simulink model "Simulink_with_unkown_parameters_case"  (R2020b)
settings: Solver=FixedStepAuto  StartTime=0.0  StopTime=50  FixedStep=0.001  MaxStep=0.01  RelTol=1e-9
values from neighbouring files (symbols this model uses):
  A0 = [30 3;3 30]    [Main_with_unkown_parameters_case.m]
  A1 = [30 3;3 30]    [Main_with_unkown_parameters_case.m]
  A2 = [10 1;1 10]    [Main_with_unkown_parameters_case.m]
  AE = blkdiag([0 pi/2;-pi/2 0],[0 pi/2;-pi/2 0])    [Main.m]    (also in Main_with_unkown_parameters_case.m)
  AM = blkdiag([0 1;-1 0],[0 1;-1 0])    [Main.m]    (also in Main_with_unkown_parameters_case.m)
  dq1_0 = [0;0]    [Main.m]    (also in Main_with_unkown_parameters_case.m)
  dq2_0 = [0;0]    [Main.m]    (also in Main_with_unkown_parameters_case.m)
  dq3_0 = [0;0]    [Main.m]    (also in Main_with_unkown_parameters_case.m)
  dq4_0 = [0;0]    [Main.m]    (also in Main_with_unkown_parameters_case.m)
  GammaE = blkdiag([1 0],[1 0])    [Main.m]    (also in Main_with_unkown_parameters_case.m)
  GammaM = blkdiag([1 0],[1 0])    [Main.m]    (also in Main_with_unkown_parameters_case.m)
  kapa = 100    [Main_with_unkown_parameters_case.m]
  Kd = 600    [Main.m]    (also in Main_with_unkown_parameters_case.m)
  Kp = 800    [Main.m]    (also in Main_with_unkown_parameters_case.m)
  l1 = 1.5    [Main.m]    (also in Main_with_unkown_parameters_case.m)
  l2 = 1.5    [Main.m]    (also in Main_with_unkown_parameters_case.m)
  M0 = [p1+p2+p4,p2;p2,p2+p5]+[2*p3,p3;p3,0]*cos(0)*0.5    [Main_with_unkown_parameters_case.m]
  N = 100    [Main_with_unkown_parameters_case.m]
  ON_OFF = 0    [Main.m]    (also in Main_with_unkown_parameters_case.m)
  p1 = m1*lc1^2+m2*l1^2+2*m2*l1*lc2^2+I1    (= 4.8375)    [Main.m]    (also in Main_with_unkown_parameters_case.m)
  p10 = 0    [Main.m]    (also in Main_with_unkown_parameters_case.m)
  p2 = m2*lc2^2+I2    (= 0.75)    [Main.m]    (also in Main_with_unkown_parameters_case.m)
  p3 = m2*l1*lc2    (= 1.125)    [Main.m]    (also in Main_with_unkown_parameters_case.m)
  p4 = 0    [Main.m]    (also in Main_with_unkown_parameters_case.m)
  p5 = 0    [Main.m]    (also in Main_with_unkown_parameters_case.m)
  p6 = (m1*lc1+m2*l1)*g    (= 23.544)    [Main.m]    (also in Main_with_unkown_parameters_case.m)
  p7 = m2*lc2*g    (= 7.3575)    [Main.m]    (also in Main_with_unkown_parameters_case.m)
  p8 = m2*lc2    (= 0.75)    [Main.m]    (also in Main_with_unkown_parameters_case.m)
  p9 = 0    [Main.m]    (also in Main_with_unkown_parameters_case.m)
  q1_0 = [-0.1;pi/3+0.2]    [Main.m]    (also in Main_with_unkown_parameters_case.m)
  q2_0 = [pi/2;2*pi/3]    [Main.m]    (also in Main_with_unkown_parameters_case.m)
  q3_0 = [pi-0.2;pi/3+0.2]    [Main.m]    (also in Main_with_unkown_parameters_case.m)
  q4_0 = [0.2;-pi/3-0.2]    [Main.m]    (also in Main_with_unkown_parameters_case.m)
  x1_0 = [0;0]    [Main.m]    (also in Main_with_unkown_parameters_case.m)
  x2_0 = [5;0]    [Main.m]    (also in Main_with_unkown_parameters_case.m)
  x3_0 = [5;3]    [Main.m]    (also in Main_with_unkown_parameters_case.m)
  x4_0 = [0;3]    [Main.m]    (also in Main_with_unkown_parameters_case.m)
(part 1 of 2)
settings Model: Creator=sokra  LastModifiedBy=sokra

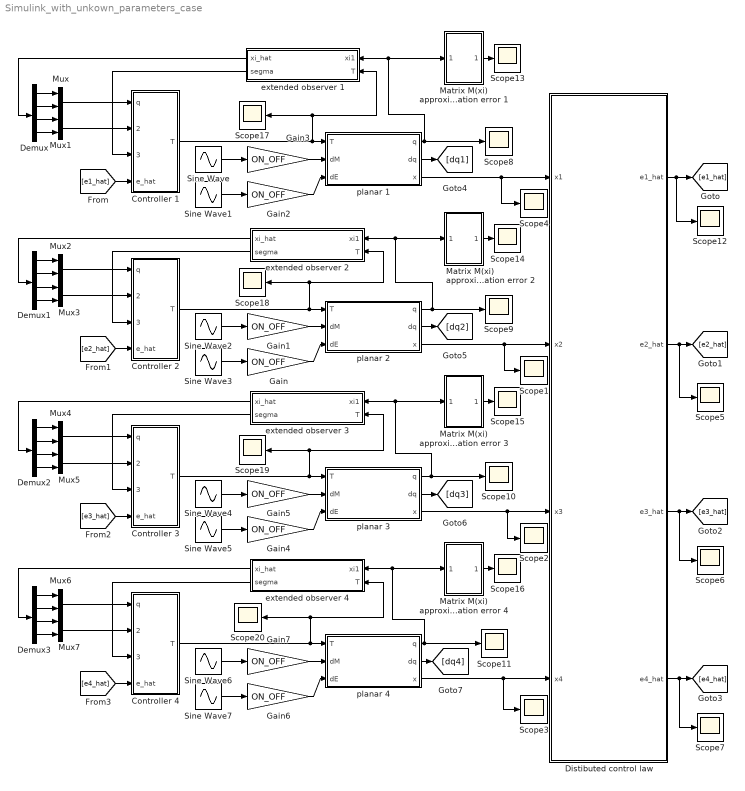
== system Simulink_with_unkown_parameters_case ==
  Controller 1 : Subsystem
  Controller 2 : Subsystem
  Controller 3 : Subsystem
  Controller 4 : Subsystem
  Demux{,1..3} (4 alike) : Demux
  Distibuted control law : MATLAB Function  TreatAsAtomicUnit=on
  Gain{,1..7} (8 alike) : Gain  Gain=ON_OFF
  Matrix M(xi) approximation error 1 : Subsystem
  Matrix M(xi) approximation error 2 : Subsystem
  Matrix M(xi) approximation error 3 : Subsystem
  Matrix M(xi) approximation error 4 : Subsystem
  Mux{,1..7} (8 alike) : Mux  Inputs=2
  Scope{1..20} (20 alike) : Scope
  Sine Wave{,2,4,6} (4 alike) : Sin  Amplitude=[1;1]  Frequency=[1;1]  SampleTime=0
  Sine Wave{1,3,5,7} (4 alike) : Sin  Amplitude=[1;1]/2  Frequency=[1;1]*pi/2  SampleTime=0
  extended observer 1 : Subsystem
  extended observer 2 : Subsystem
  extended observer 3 : Subsystem
  extended observer 4 : Subsystem
  planar 1 : Subsystem  mask{q_0=q1_0, dq_0=dq1_0, x0=x1_0}
  planar 2 : Subsystem  mask{q_0=q2_0, dq_0=dq2_0, x0=x2_0}
  planar 3 : Subsystem  mask{q_0=q3_0, dq_0=dq3_0, x0=x3_0}
  planar 4 : Subsystem  mask{q_0=q4_0, dq_0=dq4_0, x0=x4_0}
  wires:
  Controller 1/1(T) -> Scope17/1, extended observer 1/2(T), planar 1/1(T)
  planar 1/1(q) -> Scope8/1, Matrix M(xi) approximation error 1/1(xi1), extended observer 1/1(xi1)
  planar 2/1(q) -> Scope9/1, Matrix M(xi) approximation error 2/1(xi1), extended observer 2/1(xi1)
  Controller 2/1(T) -> planar 2/1(T), extended observer 2/2(T), Scope18/1
  Controller 3/1(T) -> extended observer 3/2(T), Scope19/1, planar 3/1(T)
  planar 3/1(q) -> Matrix M(xi) approximation error 3/1(xi1), extended observer 3/1(xi1), Scope10/1
  planar 4/1(q) -> Scope11/1, Matrix M(xi) approximation error 4/1(xi1), extended observer 4/1(xi1)
  Controller 4/1(T) -> extended observer 4/2(T), Scope20/1, planar 4/1(T)
  planar 1/3(x) -> Scope4/1, Distibuted control law/1(x1)
  planar 2/3(x) -> Scope1/1, Distibuted control law/2(x2)
  planar 3/3(x) -> Scope2/1, Distibuted control law/3(x3)
  planar 4/3(x) -> Scope3/1, Distibuted control law/4(x4)
  Distibuted control law/1(e1_hat) -> Scope12/1, [e1_hat]
  Distibuted control law/2(e2_hat) -> Scope5/1, [e2_hat]
  Distibuted control law/3(e3_hat) -> Scope6/1, [e3_hat]
  Distibuted control law/4(e4_hat) -> Scope7/1, [e4_hat]
  [e1_hat] -> Controller 1/4(e_hat)
  [e2_hat] -> Controller 2/4(e_hat)
  [e3_hat] -> Controller 3/4(e_hat)
  [e4_hat] -> Controller 4/4(e_hat)
  Gain/1 -> planar 2/3(dE)
  Gain1/1 -> planar 2/2(dM)
  Sine Wave2/1 -> Gain1/1
  Sine Wave3/1 -> Gain/1
  Sine Wave/1 -> Gain3/1
  Sine Wave1/1 -> Gain2/1
  Gain3/1 -> planar 1/2(dM)
  Sine Wave4/1 -> Gain5/1
  Sine Wave5/1 -> Gain4/1
  Gain5/1 -> planar 3/2(dM)
  Sine Wave6/1 -> Gain7/1
  Sine Wave7/1 -> Gain6/1
  Gain7/1 -> planar 4/2(dM)
  Gain6/1 -> planar 4/3(dE)
  Gain4/1 -> planar 3/3(dE)
  Gain2/1 -> planar 1/3(dE)
  planar 1/2(dq) -> [dq1]
  planar 2/2(dq) -> [dq2]
  planar 3/2(dq) -> [dq3]
  planar 4/2(dq) -> [dq4]
  extended observer 1/1(xi_hat) -> Demux/1
  Demux/2 -> Mux/2
  Demux/1 -> Mux/1
  Demux/3 -> Mux1/1
  Demux/4 -> Mux1/2
  Mux/1 -> Controller 1/1(q)
  Mux1/1 -> Controller 1/2(dq_hat)
  Demux1/2 -> Mux2/2
  Demux1/1 -> Mux2/1
  Demux1/4 -> Mux3/2
  Demux1/3 -> Mux3/1
  Demux2/3 -> Mux5/1
  Demux2/1 -> Mux4/1
  Demux2/4 -> Mux5/2
  Demux2/2 -> Mux4/2
  Demux3/3 -> Mux7/1
  Demux3/1 -> Mux6/1
  Demux3/4 -> Mux7/2
  Demux3/2 -> Mux6/2
  Mux2/1 -> Controller 2/1(q)
  Mux3/1 -> Controller 2/2(dq_hat)
  Mux4/1 -> Controller 3/1(q)
  Mux5/1 -> Controller 3/2(dq_hat)
  Mux6/1 -> Controller 4/1(q)
  Mux7/1 -> Controller 4/2(dq_hat)
  extended observer 4/1(xi_hat) -> Demux3/1
  extended observer 3/1(xi_hat) -> Demux2/1
  extended observer 2/1(xi_hat) -> Demux1/1
  extended observer 1/2(segma) -> Controller 1/3(segma)
  extended observer 2/2(segma) -> Controller 2/3(segma)
  extended observer 3/2(segma) -> Controller 3/3(segma)
  extended observer 4/2(segma) -> Controller 4/3(segma)
  Matrix M(xi) approximation error 1/1(error) -> Scope13/1
  Matrix M(xi) approximation error 2/1(error) -> Scope14/1
  Matrix M(xi) approximation error 3/1(error) -> Scope15/1
  Matrix M(xi) approximation error 4/1(error) -> Scope16/1

== system Simulink_with_unkown_parameters_case/Controller 1 ==
  q : Inport
  dq_hat : Inport  Port=2
  segma : Inport  Port=3
  e_hat : Inport  Port=4
  Compensator : Subsystem
  Gain1 : Gain  Gain=-Kd
  Gain2 : Gain  Gain=-Kp
  Gain3 : Gain  Gain=ON_OFF
  Gain4 : Gain  Gain=M0  Multiplication=Matrix(K*u)
  Jacobian matrix : Subsystem
  Product1 : Product  Multiplication=Matrix(*)
  Saturation : Saturate  UpperLimit=N  LowerLimit=-N
  Sum2 : Sum  Inputs=+-
  Sum5 : Sum  Inputs=+++
  Transpose : Math  Operator=transpose  SaturateOnIntegerOverflow=on
  T : Outport
  wires:
  dq_hat/1 -> Compensator/1(dq), Gain1/1
  Gain1/1 -> Sum5/3
  Sum5/1 -> Sum2/1
  Jacobian matrix/1(J(q)) -> Transpose/1
  Transpose/1 -> Compensator/2(J(q)), Gain2/1
  Gain2/1 -> Product1/1
  Product1/1 -> Sum5/2
  e_hat/1 -> Product1/2
  Compensator/1(ud) -> Gain3/1
  Gain3/1 -> Sum5/1
  q/1 -> Jacobian matrix/1(q)  "q"
  Saturation/1 -> T/1
  segma/1 -> Sum2/2
  Gain4/1 -> Saturation/1
  Sum2/1 -> Gain4/1

== system Simulink_with_unkown_parameters_case/Controller 2 ==
  q : Inport
  dq_hat : Inport  Port=2
  segma : Inport  Port=3
  e_hat : Inport  Port=4
  Compensator : Subsystem
  Gain1 : Gain  Gain=-Kd
  Gain2 : Gain  Gain=-Kp
  Gain3 : Gain  Gain=ON_OFF
  Gain4 : Gain  Gain=M0  Multiplication=Matrix(K*u)
  Jacobian matrix : Subsystem
  Product1 : Product  Multiplication=Matrix(*)
  Saturation : Saturate  UpperLimit=N  LowerLimit=-N
  Sum2 : Sum  Inputs=+-
  Sum5 : Sum  Inputs=+++
  Transpose : Math  Operator=transpose  SaturateOnIntegerOverflow=on
  T : Outport
  wires:
  dq_hat/1 -> Compensator/1(dq), Gain1/1
  Gain1/1 -> Sum5/3
  Sum5/1 -> Sum2/1
  Jacobian matrix/1(J(q)) -> Transpose/1
  Transpose/1 -> Compensator/2(J(q)), Gain2/1
  Gain2/1 -> Product1/1
  Product1/1 -> Sum5/2
  e_hat/1 -> Product1/2
  Compensator/1(ud) -> Gain3/1
  Gain3/1 -> Sum5/1
  q/1 -> Jacobian matrix/1(q)  "q"
  Saturation/1 -> T/1
  segma/1 -> Sum2/2
  Gain4/1 -> Saturation/1
  Sum2/1 -> Gain4/1

== system Simulink_with_unkown_parameters_case/Controller 3 ==
  q : Inport
  dq_hat : Inport  Port=2
  segma : Inport  Port=3
  e_hat : Inport  Port=4
  Compensator : Subsystem
  Gain1 : Gain  Gain=-Kd
  Gain2 : Gain  Gain=-Kp
  Gain3 : Gain  Gain=ON_OFF
  Gain4 : Gain  Gain=M0  Multiplication=Matrix(K*u)
  Jacobian matrix : Subsystem
  Product1 : Product  Multiplication=Matrix(*)
  Saturation : Saturate  UpperLimit=N  LowerLimit=-N
  Sum2 : Sum  Inputs=+-
  Sum5 : Sum  Inputs=+++
  Transpose : Math  Operator=transpose  SaturateOnIntegerOverflow=on
  T : Outport
  wires:
  dq_hat/1 -> Compensator/1(dq), Gain1/1
  Gain1/1 -> Sum5/3
  Sum5/1 -> Sum2/1
  Jacobian matrix/1(J(q)) -> Transpose/1
  Transpose/1 -> Compensator/2(J(q)), Gain2/1
  Gain2/1 -> Product1/1
  Product1/1 -> Sum5/2
  e_hat/1 -> Product1/2
  Compensator/1(ud) -> Gain3/1
  Gain3/1 -> Sum5/1
  q/1 -> Jacobian matrix/1(q)  "q"
  Saturation/1 -> T/1
  segma/1 -> Sum2/2
  Gain4/1 -> Saturation/1
  Sum2/1 -> Gain4/1

== system Simulink_with_unkown_parameters_case/Controller 4 ==
  q : Inport
  dq_hat : Inport  Port=2
  segma : Inport  Port=3
  e_hat : Inport  Port=4
  Compensator : Subsystem
  Gain1 : Gain  Gain=-Kd
  Gain2 : Gain  Gain=-Kp
  Gain3 : Gain  Gain=ON_OFF
  Gain4 : Gain  Gain=M0  Multiplication=Matrix(K*u)
  Jacobian matrix : Subsystem
  Product1 : Product  Multiplication=Matrix(*)
  Saturation : Saturate  UpperLimit=N  LowerLimit=-N
  Sum2 : Sum  Inputs=+-
  Sum5 : Sum  Inputs=+++
  Transpose : Math  Operator=transpose  SaturateOnIntegerOverflow=on
  T : Outport
  wires:
  dq_hat/1 -> Compensator/1(dq), Gain1/1
  Gain1/1 -> Sum5/3
  Sum5/1 -> Sum2/1
  Jacobian matrix/1(J(q)) -> Transpose/1
  Transpose/1 -> Compensator/2(J(q)), Gain2/1
  Gain2/1 -> Product1/1
  Product1/1 -> Sum5/2
  e_hat/1 -> Product1/2
  Compensator/1(ud) -> Gain3/1
  Gain3/1 -> Sum5/1
  q/1 -> Jacobian matrix/1(q)  "q"
  Saturation/1 -> T/1
  segma/1 -> Sum2/2
  Gain4/1 -> Saturation/1
  Sum2/1 -> Gain4/1

== system Simulink_with_unkown_parameters_case/Matrix M(xi) approximation error 1 ==
  xi1 : Inport
  Abs : Abs
  Constant : Constant  Value=inv(M0)
  Gain : Gain  Gain=[1;0]  Multiplication=Matrix(u*K)
  Gain1 : Gain  Gain=[0;1]  Multiplication=Matrix(u*K)
  Gain7 : Gain  Gain=M0  Multiplication=Matrix(K*u)
  "Matrix M(xi) " : Subsystem
  Max : MinMax  Function=max  Inputs=2
  Product of Elements : Product  Inputs=/  Multiplication=Matrix(*)
  Sum of Elements : Sum  Inputs=+
  Sum of Elements1 : Sum  Inputs=+
  Sum2 : Sum  Inputs=|+-
  error : Outport
  wires:
  Sum of Elements/1 -> Max/1
  Gain/1 -> Sum of Elements/1
  Gain1/1 -> Sum of Elements1/1
  Gain7/1 -> Abs/1
  Sum2/1 -> Gain7/1
  Abs/1 -> Gain/1, Gain1/1
  Sum of Elements1/1 -> Max/2
  "Matrix M(xi) "/1(M) -> Product of Elements/1
  Constant/1 -> Sum2/2
  Product of Elements/1 -> Sum2/1
  Max/1 -> error/1
  xi1/1 -> "Matrix M(xi) "/1(xi1)

== system Simulink_with_unkown_parameters_case/Matrix M(xi) approximation error 2 ==
  xi1 : Inport
  Abs : Abs
  Constant : Constant  Value=inv(M0)
  Gain : Gain  Gain=[1;0]  Multiplication=Matrix(u*K)
  Gain1 : Gain  Gain=[0;1]  Multiplication=Matrix(u*K)
  Gain7 : Gain  Gain=M0  Multiplication=Matrix(K*u)
  "Matrix M(xi) " : Subsystem
  Max : MinMax  Function=max  Inputs=2
  Product of Elements : Product  Inputs=/  Multiplication=Matrix(*)
  Sum of Elements : Sum  Inputs=+
  Sum of Elements1 : Sum  Inputs=+
  Sum2 : Sum  Inputs=|+-
  error : Outport
  wires:
  xi1/1 -> "Matrix M(xi) "/1(xi1)
  Max/1 -> error/1
  Product of Elements/1 -> Sum2/1
  Constant/1 -> Sum2/2
  "Matrix M(xi) "/1(M) -> Product of Elements/1
  Sum of Elements1/1 -> Max/2
  Abs/1 -> Gain1/1, Gain/1
  Sum2/1 -> Gain7/1
  Gain7/1 -> Abs/1
  Gain1/1 -> Sum of Elements1/1
  Gain/1 -> Sum of Elements/1
  Sum of Elements/1 -> Max/1

== system Simulink_with_unkown_parameters_case/Matrix M(xi) approximation error 3 ==
  xi1 : Inport
  Abs : Abs
  Constant : Constant  Value=inv(M0)
  Gain : Gain  Gain=[1;0]  Multiplication=Matrix(u*K)
  Gain1 : Gain  Gain=[0;1]  Multiplication=Matrix(u*K)
  Gain7 : Gain  Gain=M0  Multiplication=Matrix(K*u)
  "Matrix M(xi) " : Subsystem
  Max : MinMax  Function=max  Inputs=2
  Product of Elements : Product  Inputs=/  Multiplication=Matrix(*)
  Sum of Elements : Sum  Inputs=+
  Sum of Elements1 : Sum  Inputs=+
  Sum2 : Sum  Inputs=|+-
  error : Outport
  wires:
  xi1/1 -> "Matrix M(xi) "/1(xi1)
  Max/1 -> error/1
  Product of Elements/1 -> Sum2/1
  Constant/1 -> Sum2/2
  "Matrix M(xi) "/1(M) -> Product of Elements/1
  Sum of Elements1/1 -> Max/2
  Abs/1 -> Gain1/1, Gain/1
  Sum2/1 -> Gain7/1
  Gain7/1 -> Abs/1
  Gain1/1 -> Sum of Elements1/1
  Gain/1 -> Sum of Elements/1
  Sum of Elements/1 -> Max/1

== system Simulink_with_unkown_parameters_case/Matrix M(xi) approximation error 4 ==
  xi1 : Inport
  Abs : Abs
  Constant : Constant  Value=inv(M0)
  Gain : Gain  Gain=[1;0]  Multiplication=Matrix(u*K)
  Gain1 : Gain  Gain=[0;1]  Multiplication=Matrix(u*K)
  Gain7 : Gain  Gain=M0  Multiplication=Matrix(K*u)
  "Matrix M(xi) " : Subsystem
  Max : MinMax  Function=max  Inputs=2
  Product of Elements : Product  Inputs=/  Multiplication=Matrix(*)
  Sum of Elements : Sum  Inputs=+
  Sum of Elements1 : Sum  Inputs=+
  Sum2 : Sum  Inputs=|+-
  error : Outport
  wires:
  Sum of Elements/1 -> Max/1
  Gain/1 -> Sum of Elements/1
  Gain1/1 -> Sum of Elements1/1
  Gain7/1 -> Abs/1
  Sum2/1 -> Gain7/1
  Abs/1 -> Gain/1, Gain1/1
  Sum of Elements1/1 -> Max/2
  "Matrix M(xi) "/1(M) -> Product of Elements/1
  Constant/1 -> Sum2/2
  Product of Elements/1 -> Sum2/1
  Max/1 -> error/1
  xi1/1 -> "Matrix M(xi) "/1(xi1)

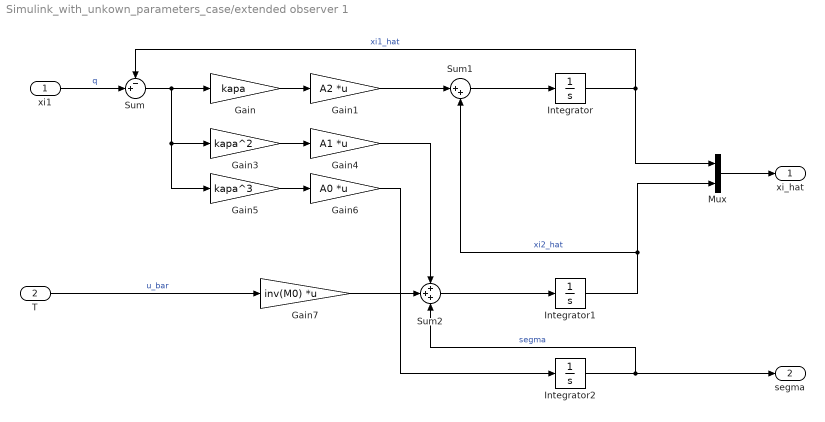
== system Simulink_with_unkown_parameters_case/extended observer 1 ==
  xi1 : Inport
  T : Inport  Port=2
  Gain : Gain  Gain=kapa
  Gain1 : Gain  Gain=A2  Multiplication=Matrix(K*u)
  Gain3 : Gain  Gain=kapa^2
  Gain4 : Gain  Gain=A1  Multiplication=Matrix(K*u)
  Gain5 : Gain  Gain=kapa^3
  Gain6 : Gain  Gain=A0  Multiplication=Matrix(K*u)
  Gain7 : Gain  Gain=inv(M0)  Multiplication=Matrix(K*u)
  Integrator : Integrator  InitialCondition=[0;0]
  Integrator1 : Integrator  InitialCondition=[0;0]
  Integrator2 : Integrator  InitialCondition=[0;0]
  Mux : Mux  Inputs=2
  Sum : Sum  Inputs=-+|
  Sum1 : Sum  Inputs=|++
  Sum2 : Sum  Inputs=+++
  xi_hat : Outport
  segma : Outport  Port=2
  wires:
  Mux/1 -> xi_hat/1
  Integrator1/1 -> Mux/2, Sum1/2  "xi2_hat"
  Integrator2/1 -> segma/1, Sum2/3  "segma"
  Integrator/1 -> Mux/1, Sum/1  "xi1_hat"
  Sum1/1 -> Integrator/1
  Gain/1 -> Gain1/1
  xi1/1 -> Sum/2  "q"
  Sum/1 -> Gain5/1, Gain3/1, Gain/1
  Gain1/1 -> Sum1/1
  T/1 -> Gain7/1  "u_bar"
  Gain3/1 -> Gain4/1
  Gain5/1 -> Gain6/1
  Gain7/1 -> Sum2/2
  Gain4/1 -> Sum2/1
  Sum2/1 -> Integrator1/1
  Gain6/1 -> Integrator2/1

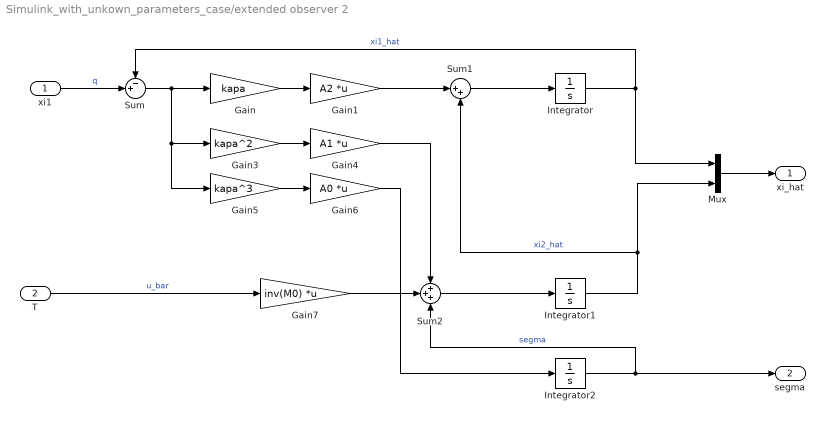
== system Simulink_with_unkown_parameters_case/extended observer 2 ==
  xi1 : Inport
  T : Inport  Port=2
  Gain : Gain  Gain=kapa
  Gain1 : Gain  Gain=A2  Multiplication=Matrix(K*u)
  Gain3 : Gain  Gain=kapa^2
  Gain4 : Gain  Gain=A1  Multiplication=Matrix(K*u)
  Gain5 : Gain  Gain=kapa^3
  Gain6 : Gain  Gain=A0  Multiplication=Matrix(K*u)
  Gain7 : Gain  Gain=inv(M0)  Multiplication=Matrix(K*u)
  Integrator : Integrator  InitialCondition=[0;0]
  Integrator1 : Integrator  InitialCondition=[0;0]
  Integrator2 : Integrator  InitialCondition=[0;0]
  Mux : Mux  Inputs=2
  Sum : Sum  Inputs=-+|
  Sum1 : Sum  Inputs=|++
  Sum2 : Sum  Inputs=+++
  xi_hat : Outport
  segma : Outport  Port=2
  wires:
  Mux/1 -> xi_hat/1
  Integrator1/1 -> Mux/2, Sum1/2  "xi2_hat"
  Integrator2/1 -> segma/1, Sum2/3  "segma"
  Integrator/1 -> Mux/1, Sum/1  "xi1_hat"
  Sum1/1 -> Integrator/1
  Gain/1 -> Gain1/1
  xi1/1 -> Sum/2  "q"
  Sum/1 -> Gain5/1, Gain3/1, Gain/1
  Gain1/1 -> Sum1/1
  T/1 -> Gain7/1  "u_bar"
  Gain3/1 -> Gain4/1
  Gain5/1 -> Gain6/1
  Gain7/1 -> Sum2/2
  Gain4/1 -> Sum2/1
  Sum2/1 -> Integrator1/1
  Gain6/1 -> Integrator2/1

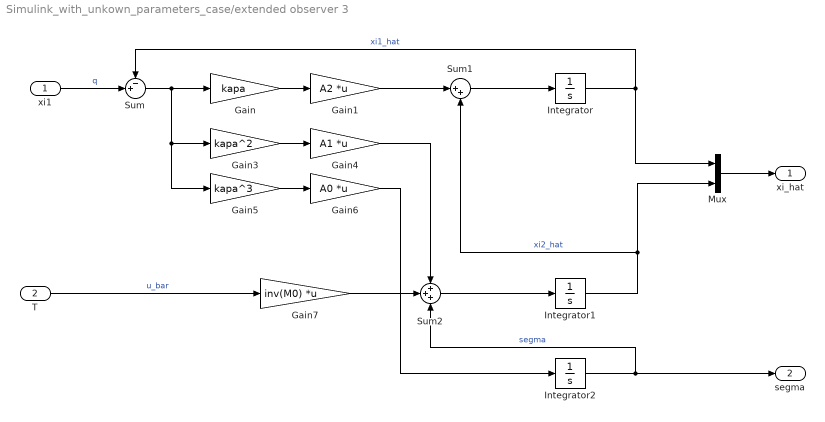
== system Simulink_with_unkown_parameters_case/extended observer 3 ==
  xi1 : Inport
  T : Inport  Port=2
  Gain : Gain  Gain=kapa
  Gain1 : Gain  Gain=A2  Multiplication=Matrix(K*u)
  Gain3 : Gain  Gain=kapa^2
  Gain4 : Gain  Gain=A1  Multiplication=Matrix(K*u)
  Gain5 : Gain  Gain=kapa^3
  Gain6 : Gain  Gain=A0  Multiplication=Matrix(K*u)
  Gain7 : Gain  Gain=inv(M0)  Multiplication=Matrix(K*u)
  Integrator : Integrator  InitialCondition=[0;0]
  Integrator1 : Integrator  InitialCondition=[0;0]
  Integrator2 : Integrator  InitialCondition=[0;0]
  Mux : Mux  Inputs=2
  Sum : Sum  Inputs=-+|
  Sum1 : Sum  Inputs=|++
  Sum2 : Sum  Inputs=+++
  xi_hat : Outport
  segma : Outport  Port=2
  wires:
  Mux/1 -> xi_hat/1
  Integrator1/1 -> Mux/2, Sum1/2  "xi2_hat"
  Integrator2/1 -> segma/1, Sum2/3  "segma"
  Integrator/1 -> Mux/1, Sum/1  "xi1_hat"
  Sum1/1 -> Integrator/1
  Gain/1 -> Gain1/1
  xi1/1 -> Sum/2  "q"
  Sum/1 -> Gain5/1, Gain3/1, Gain/1
  Gain1/1 -> Sum1/1
  T/1 -> Gain7/1  "u_bar"
  Gain3/1 -> Gain4/1
  Gain5/1 -> Gain6/1
  Gain7/1 -> Sum2/2
  Gain4/1 -> Sum2/1
  Sum2/1 -> Integrator1/1
  Gain6/1 -> Integrator2/1

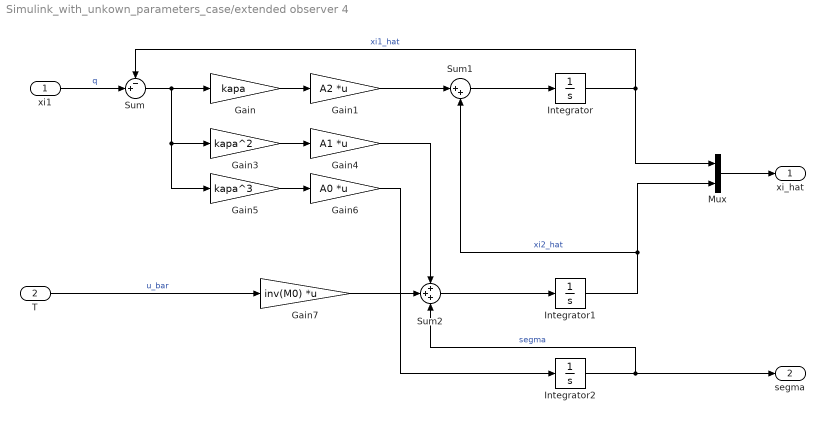
== system Simulink_with_unkown_parameters_case/extended observer 4 ==
  xi1 : Inport
  T : Inport  Port=2
  Gain : Gain  Gain=kapa
  Gain1 : Gain  Gain=A2  Multiplication=Matrix(K*u)
  Gain3 : Gain  Gain=kapa^2
  Gain4 : Gain  Gain=A1  Multiplication=Matrix(K*u)
  Gain5 : Gain  Gain=kapa^3
  Gain6 : Gain  Gain=A0  Multiplication=Matrix(K*u)
  Gain7 : Gain  Gain=inv(M0)  Multiplication=Matrix(K*u)
  Integrator : Integrator  InitialCondition=[0;0]
  Integrator1 : Integrator  InitialCondition=[0;0]
  Integrator2 : Integrator  InitialCondition=[0;0]
  Mux : Mux  Inputs=2
  Sum : Sum  Inputs=-+|
  Sum1 : Sum  Inputs=|++
  Sum2 : Sum  Inputs=+++
  xi_hat : Outport
  segma : Outport  Port=2
  wires:
  Mux/1 -> xi_hat/1
  Integrator1/1 -> Mux/2, Sum1/2  "xi2_hat"
  Integrator2/1 -> segma/1, Sum2/3  "segma"
  Integrator/1 -> Mux/1, Sum/1  "xi1_hat"
  Sum1/1 -> Integrator/1
  Gain/1 -> Gain1/1
  xi1/1 -> Sum/2  "q"
  Sum/1 -> Gain5/1, Gain3/1, Gain/1
  Gain1/1 -> Sum1/1
  T/1 -> Gain7/1  "u_bar"
  Gain3/1 -> Gain4/1
  Gain5/1 -> Gain6/1
  Gain7/1 -> Sum2/2
  Gain4/1 -> Sum2/1
  Sum2/1 -> Integrator1/1
  Gain6/1 -> Integrator2/1

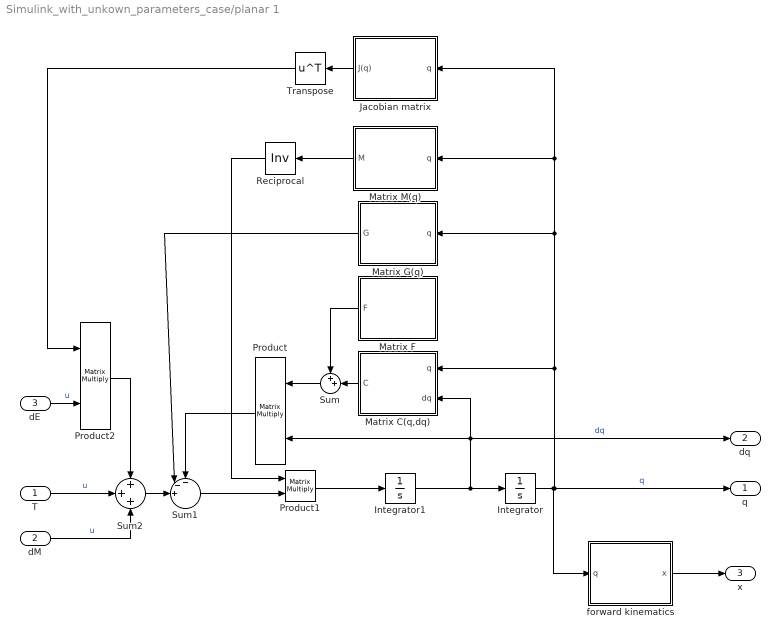
== system Simulink_with_unkown_parameters_case/planar 1 ==
  T : Inport
  dM : Inport  Port=2
  dE : Inport  Port=3
  Integrator : Integrator  InitialCondition=q_0
  Integrator1 : Integrator  InitialCondition=dq_0
  Jacobian matrix : Subsystem
  "Matrix C(q,dq) " : Subsystem
  Matrix F : Subsystem
  Matrix G(q) : Subsystem
  "Matrix M(q) " : Subsystem
  Product : Product  Multiplication=Matrix(*)
  Product1 : Product  Multiplication=Matrix(*)
  Product2 : Product  Multiplication=Matrix(*)
  Reciprocal : Product  Inputs=/  Multiplication=Matrix(*)
  Sum : Sum  Inputs=++|
  Sum1 : Sum  Inputs=--+||
  Sum2 : Sum  Inputs=+++
  Transpose : Math  Operator=transpose  SaturateOnIntegerOverflow=on
  forward kinematics : Subsystem
  q : Outport
  dq : Outport  Port=2
  x : Outport  Port=3
  wires:
  Jacobian matrix/1(J(q)) -> Transpose/1
  Transpose/1 -> Product2/1
  Integrator/1 -> q/1, "Matrix C(q,dq) "/1(q), Matrix G(q)/1(q), Jacobian matrix/1(q), "Matrix M(q) "/1(q), forward kinematics/1(q)  "q"
  Matrix G(q)/1(G) -> Sum1/2
  dE/1 -> Product2/2  "u"
  Product1/1 -> Integrator1/1
  Matrix F/1(F) -> Sum/1
  Reciprocal/1 -> Product1/1
  Integrator1/1 -> Product/2, "Matrix C(q,dq) "/2(dq), dq/1, Integrator/1  "dq"
  "Matrix C(q,dq) "/1(C) -> Sum/2
  Product/1 -> Sum1/1
  "Matrix M(q) "/1(M) -> Reciprocal/1
  Sum1/1 -> Product1/2
  T/1 -> Sum2/2  "u"
  dM/1 -> Sum2/3  "u"
  Sum2/1 -> Sum1/3
  Product2/1 -> Sum2/1
  forward kinematics/1(x) -> x/1
  Sum/1 -> Product/1

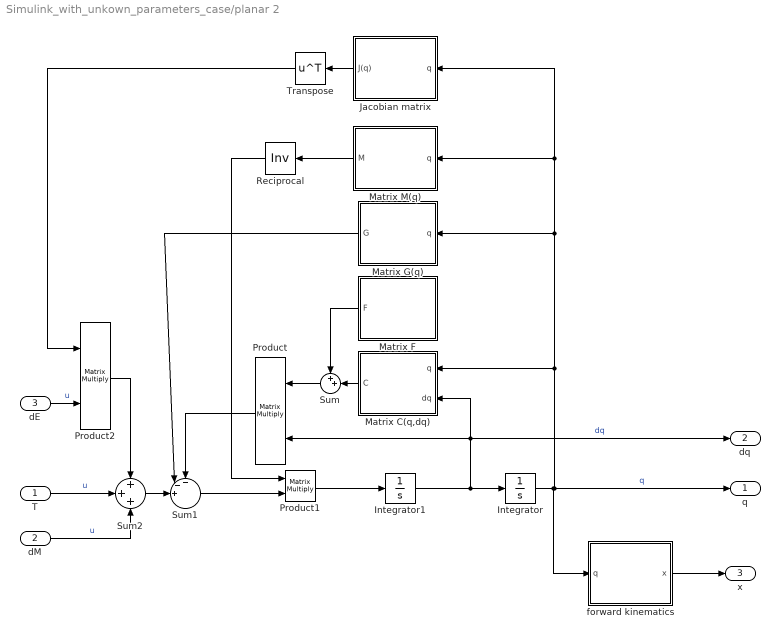
== system Simulink_with_unkown_parameters_case/planar 2 ==
  T : Inport
  dM : Inport  Port=2
  dE : Inport  Port=3
  Integrator : Integrator  InitialCondition=q_0
  Integrator1 : Integrator  InitialCondition=dq_0
  Jacobian matrix : Subsystem
  "Matrix C(q,dq) " : Subsystem
  Matrix F : Subsystem
  Matrix G(q) : Subsystem
  "Matrix M(q) " : Subsystem
  Product : Product  Multiplication=Matrix(*)
  Product1 : Product  Multiplication=Matrix(*)
  Product2 : Product  Multiplication=Matrix(*)
  Reciprocal : Product  Inputs=/  Multiplication=Matrix(*)
  Sum : Sum  Inputs=++|
  Sum1 : Sum  Inputs=--+||
  Sum2 : Sum  Inputs=+++
  Transpose : Math  Operator=transpose  SaturateOnIntegerOverflow=on
  forward kinematics : Subsystem
  q : Outport
  dq : Outport  Port=2
  x : Outport  Port=3
  wires:
  forward kinematics/1(x) -> x/1
  Matrix G(q)/1(G) -> Sum1/2
  Product/1 -> Sum1/1
  Reciprocal/1 -> Product1/1
  Sum1/1 -> Product1/2
  Sum/1 -> Product/1
  "Matrix C(q,dq) "/1(C) -> Sum/2
  Integrator1/1 -> Product/2, "Matrix C(q,dq) "/2(dq), dq/1, Integrator/1  "dq"
  Product1/1 -> Integrator1/1
  Matrix F/1(F) -> Sum/1
  Sum2/1 -> Sum1/3
  "Matrix M(q) "/1(M) -> Reciprocal/1
  T/1 -> Sum2/2  "u"
  dM/1 -> Sum2/3  "u"
  Transpose/1 -> Product2/1
  Jacobian matrix/1(J(q)) -> Transpose/1
  Integrator/1 -> q/1, "Matrix C(q,dq) "/1(q), Matrix G(q)/1(q), Jacobian matrix/1(q), "Matrix M(q) "/1(q), forward kinematics/1(q)  "q"
  Product2/1 -> Sum2/1
  dE/1 -> Product2/2  "u"

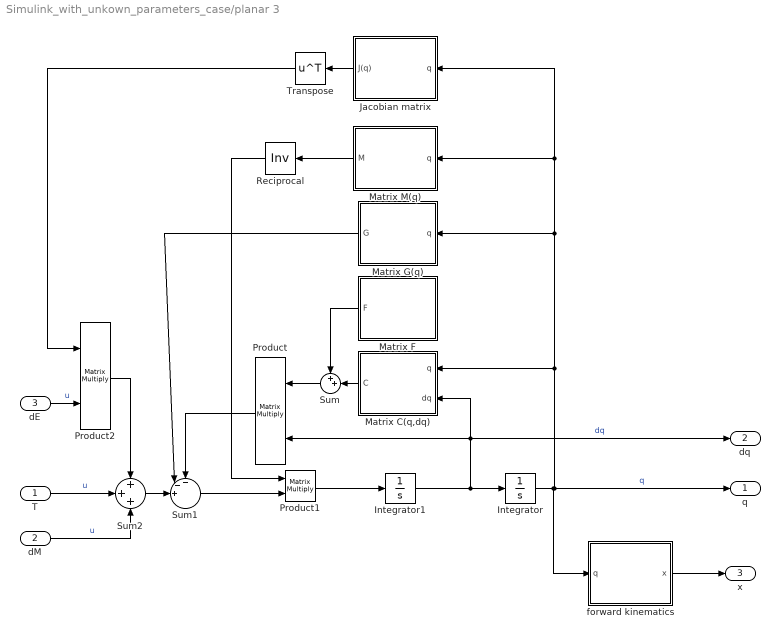
== system Simulink_with_unkown_parameters_case/planar 3 ==
  T : Inport
  dM : Inport  Port=2
  dE : Inport  Port=3
  Integrator : Integrator  InitialCondition=q_0
  Integrator1 : Integrator  InitialCondition=dq_0
  Jacobian matrix : Subsystem
  "Matrix C(q,dq) " : Subsystem
  Matrix F : Subsystem
  Matrix G(q) : Subsystem
  "Matrix M(q) " : Subsystem
  Product : Product  Multiplication=Matrix(*)
  Product1 : Product  Multiplication=Matrix(*)
  Product2 : Product  Multiplication=Matrix(*)
  Reciprocal : Product  Inputs=/  Multiplication=Matrix(*)
  Sum : Sum  Inputs=++|
  Sum1 : Sum  Inputs=--+||
  Sum2 : Sum  Inputs=+++
  Transpose : Math  Operator=transpose  SaturateOnIntegerOverflow=on
  forward kinematics : Subsystem
  q : Outport
  dq : Outport  Port=2
  x : Outport  Port=3
  wires:
  Jacobian matrix/1(J(q)) -> Transpose/1
  Transpose/1 -> Product2/1
  Integrator/1 -> q/1, "Matrix C(q,dq) "/1(q), Matrix G(q)/1(q), Jacobian matrix/1(q), "Matrix M(q) "/1(q), forward kinematics/1(q)  "q"
  Matrix G(q)/1(G) -> Sum1/2
  dE/1 -> Product2/2  "u"
  Product1/1 -> Integrator1/1
  Matrix F/1(F) -> Sum/1
  Reciprocal/1 -> Product1/1
  Integrator1/1 -> Product/2, "Matrix C(q,dq) "/2(dq), dq/1, Integrator/1  "dq"
  "Matrix C(q,dq) "/1(C) -> Sum/2
  Product/1 -> Sum1/1
  "Matrix M(q) "/1(M) -> Reciprocal/1
  Sum1/1 -> Product1/2
  T/1 -> Sum2/2  "u"
  dM/1 -> Sum2/3  "u"
  Sum2/1 -> Sum1/3
  Product2/1 -> Sum2/1
  forward kinematics/1(x) -> x/1
  Sum/1 -> Product/1

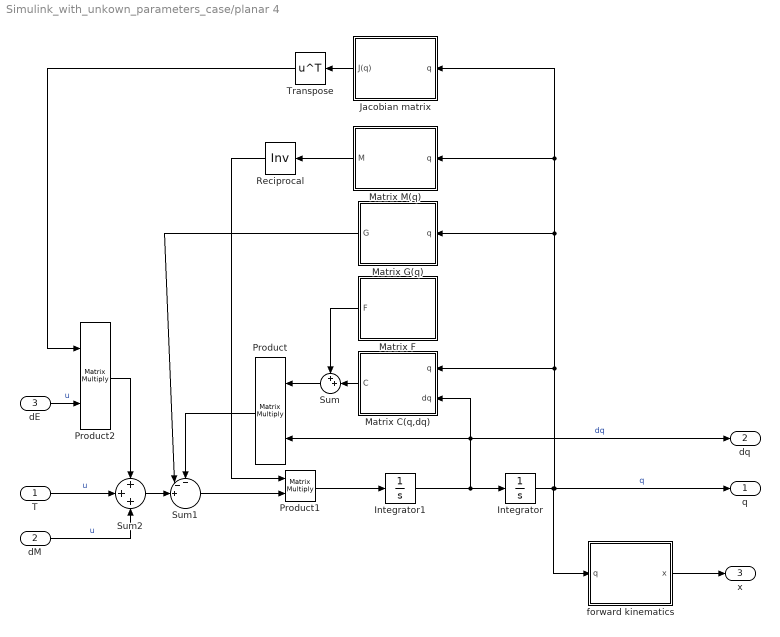
== system Simulink_with_unkown_parameters_case/planar 4 ==
  T : Inport
  dM : Inport  Port=2
  dE : Inport  Port=3
  Integrator : Integrator  InitialCondition=q_0
  Integrator1 : Integrator  InitialCondition=dq_0
  Jacobian matrix : Subsystem
  "Matrix C(q,dq) " : Subsystem
  Matrix F : Subsystem
  Matrix G(q) : Subsystem
  "Matrix M(q) " : Subsystem
  Product : Product  Multiplication=Matrix(*)
  Product1 : Product  Multiplication=Matrix(*)
  Product2 : Product  Multiplication=Matrix(*)
  Reciprocal : Product  Inputs=/  Multiplication=Matrix(*)
  Sum : Sum  Inputs=++|
  Sum1 : Sum  Inputs=--+||
  Sum2 : Sum  Inputs=+++
  Transpose : Math  Operator=transpose  SaturateOnIntegerOverflow=on
  forward kinematics : Subsystem
  q : Outport
  dq : Outport  Port=2
  x : Outport  Port=3
  wires:
  Jacobian matrix/1(J(q)) -> Transpose/1
  Transpose/1 -> Product2/1
  Integrator/1 -> q/1, "Matrix C(q,dq) "/1(q), Matrix G(q)/1(q), Jacobian matrix/1(q), "Matrix M(q) "/1(q), forward kinematics/1(q)  "q"
  Matrix G(q)/1(G) -> Sum1/2
  dE/1 -> Product2/2  "u"
  Product1/1 -> Integrator1/1
  Matrix F/1(F) -> Sum/1
  Reciprocal/1 -> Product1/1
  Integrator1/1 -> Product/2, "Matrix C(q,dq) "/2(dq), dq/1, Integrator/1  "dq"
  "Matrix C(q,dq) "/1(C) -> Sum/2
  Product/1 -> Sum1/1
  "Matrix M(q) "/1(M) -> Reciprocal/1
  Sum1/1 -> Product1/2
  T/1 -> Sum2/2  "u"
  dM/1 -> Sum2/3  "u"
  Sum2/1 -> Sum1/3
  Product2/1 -> Sum2/1
  forward kinematics/1(x) -> x/1
  Sum/1 -> Product/1

== system Simulink_with_unkown_parameters_case/Controller 1/Compensator ==
  dq : Inport
  J(q) : Inport  Port=2
  Gain : Gain  Gain=AM  Multiplication=Matrix(K*u)
  Gain3 : Gain  Gain=GammaM'  Multiplication=Matrix(K*u)
  Gain4 : Gain  Gain=GammaM  Multiplication=Matrix(K*u)
  Gain5 : Gain  Gain=AE  Multiplication=Matrix(K*u)
  Gain6 : Gain  Gain=GammaE'  Multiplication=Matrix(K*u)
  Gain7 : Gain  Gain=GammaE  Multiplication=Matrix(K*u)
  Integrator : Integrator  InitialCondition=[0;0;0;0]
  Integrator1 : Integrator  InitialCondition=[0;0;0;0]
  Product1 : Product  Multiplication=Matrix(*)
  Product2 : Product  Multiplication=Matrix(*)
  Sum1 : Sum
  Sum2 : Sum  Inputs=|-+
  Sum3 : Sum  Inputs=|-+
  ud : Outport
  wires:
  Product2/1 -> Gain6/1
  Integrator/1 -> Gain4/1, Gain/1
  Gain3/1 -> Sum2/1
  Gain/1 -> Sum2/2
  Sum3/1 -> Integrator1/1
  Gain5/1 -> Sum3/2
  Sum2/1 -> Integrator/1
  dq/1 -> Gain3/1, Product2/2
  Gain6/1 -> Sum3/1
  Sum1/1 -> ud/1
  Gain4/1 -> Sum1/1
  Product1/1 -> Sum1/2
  J(q)/1 -> Product1/1, Product2/1
  Gain7/1 -> Product1/2
  Integrator1/1 -> Gain7/1, Gain5/1

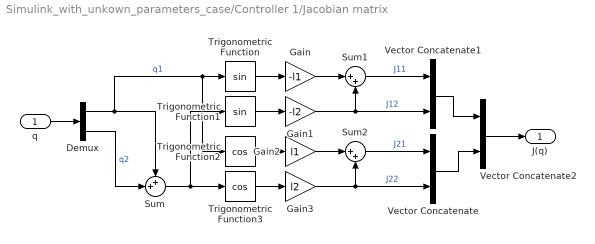
== system Simulink_with_unkown_parameters_case/Controller 1/Jacobian matrix ==
  q : Inport
  Demux : Demux  Outputs=2
  Gain : Gain  Gain=-l1
  Gain1 : Gain  Gain=-l2
  Gain2 : Gain  Gain=l1
  Gain3 : Gain  Gain=l2
  Sum : Sum  Inputs=++|
  Sum1 : Sum  Inputs=|++
  Sum2 : Sum  Inputs=|++
  Trigonometric Function : Trigonometry
  Trigonometric Function1 : Trigonometry
  Trigonometric Function2 : Trigonometry  Operator=cos
  Trigonometric Function3 : Trigonometry  Operator=cos
  Vector Concatenate : Concatenate  Mode=Multidimensional array  ConcatenateDimension=2
  Vector Concatenate1 : Concatenate  Mode=Multidimensional array  ConcatenateDimension=2
  Vector Concatenate2 : Concatenate  Mode=Multidimensional array
  J(q) : Outport
  wires:
  q/1 -> Demux/1
  Demux/2 -> Sum/2  "q2"
  Trigonometric Function/1 -> Gain/1
  Demux/1 -> Sum/1, Trigonometric Function/1, Trigonometric Function2/1  "q1"
  Sum/1 -> Trigonometric Function1/1, Trigonometric Function3/1
  Trigonometric Function1/1 -> Gain1/1
  Trigonometric Function3/1 -> Gain3/1
  Trigonometric Function2/1 -> Gain2/1
  Gain1/1 -> Vector Concatenate1/2, Sum1/2  "J12"
  Gain/1 -> Sum1/1
  Gain2/1 -> Sum2/1
  Gain3/1 -> Sum2/2, Vector Concatenate/2  "J22"
  Sum1/1 -> Vector Concatenate1/1  "J11"
  Sum2/1 -> Vector Concatenate/1  "J21"
  Vector Concatenate1/1 -> Vector Concatenate2/1
  Vector Concatenate/1 -> Vector Concatenate2/2
  Vector Concatenate2/1 -> J(q)/1

== system Simulink_with_unkown_parameters_case/Controller 2/Compensator ==
  dq : Inport
  J(q) : Inport  Port=2
  Gain : Gain  Gain=AM  Multiplication=Matrix(K*u)
  Gain3 : Gain  Gain=GammaM'  Multiplication=Matrix(K*u)
  Gain4 : Gain  Gain=GammaM  Multiplication=Matrix(K*u)
  Gain5 : Gain  Gain=AE  Multiplication=Matrix(K*u)
  Gain6 : Gain  Gain=GammaE'  Multiplication=Matrix(K*u)
  Gain7 : Gain  Gain=GammaE  Multiplication=Matrix(K*u)
  Integrator : Integrator  InitialCondition=[0;0;0;0]
  Integrator1 : Integrator  InitialCondition=[0;0;0;0]
  Product1 : Product  Multiplication=Matrix(*)
  Product2 : Product  Multiplication=Matrix(*)
  Sum1 : Sum
  Sum2 : Sum  Inputs=|-+
  Sum3 : Sum  Inputs=|-+
  ud : Outport
  wires:
  Product2/1 -> Gain6/1
  Integrator/1 -> Gain4/1, Gain/1
  Gain3/1 -> Sum2/1
  Gain/1 -> Sum2/2
  Sum3/1 -> Integrator1/1
  Gain5/1 -> Sum3/2
  Sum2/1 -> Integrator/1
  dq/1 -> Gain3/1, Product2/2
  Gain6/1 -> Sum3/1
  Sum1/1 -> ud/1
  Gain4/1 -> Sum1/1
  Product1/1 -> Sum1/2
  J(q)/1 -> Product1/1, Product2/1
  Gain7/1 -> Product1/2
  Integrator1/1 -> Gain7/1, Gain5/1

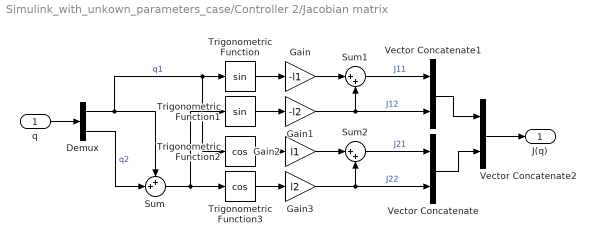
== system Simulink_with_unkown_parameters_case/Controller 2/Jacobian matrix ==
  q : Inport
  Demux : Demux  Outputs=2
  Gain : Gain  Gain=-l1
  Gain1 : Gain  Gain=-l2
  Gain2 : Gain  Gain=l1
  Gain3 : Gain  Gain=l2
  Sum : Sum  Inputs=++|
  Sum1 : Sum  Inputs=|++
  Sum2 : Sum  Inputs=|++
  Trigonometric Function : Trigonometry
  Trigonometric Function1 : Trigonometry
  Trigonometric Function2 : Trigonometry  Operator=cos
  Trigonometric Function3 : Trigonometry  Operator=cos
  Vector Concatenate : Concatenate  Mode=Multidimensional array  ConcatenateDimension=2
  Vector Concatenate1 : Concatenate  Mode=Multidimensional array  ConcatenateDimension=2
  Vector Concatenate2 : Concatenate  Mode=Multidimensional array
  J(q) : Outport
  wires:
  q/1 -> Demux/1
  Demux/2 -> Sum/2  "q2"
  Trigonometric Function/1 -> Gain/1
  Demux/1 -> Sum/1, Trigonometric Function/1, Trigonometric Function2/1  "q1"
  Sum/1 -> Trigonometric Function1/1, Trigonometric Function3/1
  Trigonometric Function1/1 -> Gain1/1
  Trigonometric Function3/1 -> Gain3/1
  Trigonometric Function2/1 -> Gain2/1
  Gain1/1 -> Vector Concatenate1/2, Sum1/2  "J12"
  Gain/1 -> Sum1/1
  Gain2/1 -> Sum2/1
  Gain3/1 -> Sum2/2, Vector Concatenate/2  "J22"
  Sum1/1 -> Vector Concatenate1/1  "J11"
  Sum2/1 -> Vector Concatenate/1  "J21"
  Vector Concatenate1/1 -> Vector Concatenate2/1
  Vector Concatenate/1 -> Vector Concatenate2/2
  Vector Concatenate2/1 -> J(q)/1

== system Simulink_with_unkown_parameters_case/Controller 3/Compensator ==
  dq : Inport
  J(q) : Inport  Port=2
  Gain : Gain  Gain=AM  Multiplication=Matrix(K*u)
  Gain3 : Gain  Gain=GammaM'  Multiplication=Matrix(K*u)
  Gain4 : Gain  Gain=GammaM  Multiplication=Matrix(K*u)
  Gain5 : Gain  Gain=AE  Multiplication=Matrix(K*u)
  Gain6 : Gain  Gain=GammaE'  Multiplication=Matrix(K*u)
  Gain7 : Gain  Gain=GammaE  Multiplication=Matrix(K*u)
  Integrator : Integrator  InitialCondition=[0;0;0;0]
  Integrator1 : Integrator  InitialCondition=[0;0;0;0]
  Product1 : Product  Multiplication=Matrix(*)
  Product2 : Product  Multiplication=Matrix(*)
  Sum1 : Sum
  Sum2 : Sum  Inputs=|-+
  Sum3 : Sum  Inputs=|-+
  ud : Outport
  wires:
  Product2/1 -> Gain6/1
  Integrator/1 -> Gain4/1, Gain/1
  Gain3/1 -> Sum2/1
  Gain/1 -> Sum2/2
  Sum3/1 -> Integrator1/1
  Gain5/1 -> Sum3/2
  Sum2/1 -> Integrator/1
  dq/1 -> Gain3/1, Product2/2
  Gain6/1 -> Sum3/1
  Sum1/1 -> ud/1
  Gain4/1 -> Sum1/1
  Product1/1 -> Sum1/2
  J(q)/1 -> Product1/1, Product2/1
  Gain7/1 -> Product1/2
  Integrator1/1 -> Gain7/1, Gain5/1

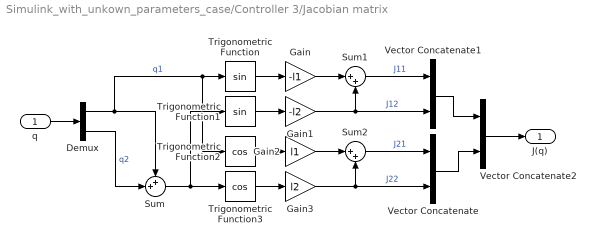
== system Simulink_with_unkown_parameters_case/Controller 3/Jacobian matrix ==
  q : Inport
  Demux : Demux  Outputs=2
  Gain : Gain  Gain=-l1
  Gain1 : Gain  Gain=-l2
  Gain2 : Gain  Gain=l1
  Gain3 : Gain  Gain=l2
  Sum : Sum  Inputs=++|
  Sum1 : Sum  Inputs=|++
  Sum2 : Sum  Inputs=|++
  Trigonometric Function : Trigonometry
  Trigonometric Function1 : Trigonometry
  Trigonometric Function2 : Trigonometry  Operator=cos
  Trigonometric Function3 : Trigonometry  Operator=cos
  Vector Concatenate : Concatenate  Mode=Multidimensional array  ConcatenateDimension=2
  Vector Concatenate1 : Concatenate  Mode=Multidimensional array  ConcatenateDimension=2
  Vector Concatenate2 : Concatenate  Mode=Multidimensional array
  J(q) : Outport
  wires:
  q/1 -> Demux/1
  Demux/2 -> Sum/2  "q2"
  Trigonometric Function/1 -> Gain/1
  Demux/1 -> Sum/1, Trigonometric Function/1, Trigonometric Function2/1  "q1"
  Sum/1 -> Trigonometric Function1/1, Trigonometric Function3/1
  Trigonometric Function1/1 -> Gain1/1
  Trigonometric Function3/1 -> Gain3/1
  Trigonometric Function2/1 -> Gain2/1
  Gain1/1 -> Vector Concatenate1/2, Sum1/2  "J12"
  Gain/1 -> Sum1/1
  Gain2/1 -> Sum2/1
  Gain3/1 -> Sum2/2, Vector Concatenate/2  "J22"
  Sum1/1 -> Vector Concatenate1/1  "J11"
  Sum2/1 -> Vector Concatenate/1  "J21"
  Vector Concatenate1/1 -> Vector Concatenate2/1
  Vector Concatenate/1 -> Vector Concatenate2/2
  Vector Concatenate2/1 -> J(q)/1

== system Simulink_with_unkown_parameters_case/Controller 4/Compensator ==
  dq : Inport
  J(q) : Inport  Port=2
  Gain : Gain  Gain=AM  Multiplication=Matrix(K*u)
  Gain3 : Gain  Gain=GammaM'  Multiplication=Matrix(K*u)
  Gain4 : Gain  Gain=GammaM  Multiplication=Matrix(K*u)
  Gain5 : Gain  Gain=AE  Multiplication=Matrix(K*u)
  Gain6 : Gain  Gain=GammaE'  Multiplication=Matrix(K*u)
  Gain7 : Gain  Gain=GammaE  Multiplication=Matrix(K*u)
  Integrator : Integrator  InitialCondition=[0;0;0;0]
  Integrator1 : Integrator  InitialCondition=[0;0;0;0]
  Product1 : Product  Multiplication=Matrix(*)
  Product2 : Product  Multiplication=Matrix(*)
  Sum1 : Sum
  Sum2 : Sum  Inputs=|-+
  Sum3 : Sum  Inputs=|-+
  ud : Outport
  wires:
  Product2/1 -> Gain6/1
  Integrator/1 -> Gain4/1, Gain/1
  Gain3/1 -> Sum2/1
  Gain/1 -> Sum2/2
  Sum3/1 -> Integrator1/1
  Gain5/1 -> Sum3/2
  Sum2/1 -> Integrator/1
  dq/1 -> Gain3/1, Product2/2
  Gain6/1 -> Sum3/1
  Sum1/1 -> ud/1
  Gain4/1 -> Sum1/1
  Product1/1 -> Sum1/2
  J(q)/1 -> Product1/1, Product2/1
  Gain7/1 -> Product1/2
  Integrator1/1 -> Gain7/1, Gain5/1

== system Simulink_with_unkown_parameters_case/Controller 4/Jacobian matrix ==
  q : Inport
  Demux : Demux  Outputs=2
  Gain : Gain  Gain=-l1
  Gain1 : Gain  Gain=-l2
  Gain2 : Gain  Gain=l1
  Gain3 : Gain  Gain=l2
  Sum : Sum  Inputs=++|
  Sum1 : Sum  Inputs=|++
  Sum2 : Sum  Inputs=|++
  Trigonometric Function : Trigonometry
  Trigonometric Function1 : Trigonometry
  Trigonometric Function2 : Trigonometry  Operator=cos
  Trigonometric Function3 : Trigonometry  Operator=cos
  Vector Concatenate : Concatenate  Mode=Multidimensional array  ConcatenateDimension=2
  Vector Concatenate1 : Concatenate  Mode=Multidimensional array  ConcatenateDimension=2
  Vector Concatenate2 : Concatenate  Mode=Multidimensional array
  J(q) : Outport
  wires:
  q/1 -> Demux/1
  Demux/2 -> Sum/2  "q2"
  Trigonometric Function/1 -> Gain/1
  Demux/1 -> Sum/1, Trigonometric Function/1, Trigonometric Function2/1  "q1"
  Sum/1 -> Trigonometric Function1/1, Trigonometric Function3/1
  Trigonometric Function1/1 -> Gain1/1
  Trigonometric Function3/1 -> Gain3/1
  Trigonometric Function2/1 -> Gain2/1
  Gain1/1 -> Vector Concatenate1/2, Sum1/2  "J12"
  Gain/1 -> Sum1/1
  Gain2/1 -> Sum2/1
  Gain3/1 -> Sum2/2, Vector Concatenate/2  "J22"
  Sum1/1 -> Vector Concatenate1/1  "J11"
  Sum2/1 -> Vector Concatenate/1  "J21"
  Vector Concatenate1/1 -> Vector Concatenate2/1
  Vector Concatenate/1 -> Vector Concatenate2/2
  Vector Concatenate2/1 -> J(q)/1

== system Simulink_with_unkown_parameters_case/Matrix M(xi) approximation error 1/Matrix M(xi)  ==
  xi1 : Inport
  Constant : Constant  Value=[p1+p2+p4,p2;p2,p2+p5]
  Demux : Demux  Outputs=2
  Gain : Gain  Gain=[2*p3,p3;p3,0]
  Sum : Sum  Inputs=|++
  Terminator : Terminator
  Trigonometric Function : Trigonometry  Operator=cos
  Vector Concatenate : Concatenate  Mode=Multidimensional array
  Vector Concatenate1 : Concatenate  Mode=Multidimensional array  ConcatenateDimension=2
  M : Outport
  wires:
  Gain/1 -> Sum/2
  Trigonometric Function/1 -> Vector Concatenate/1, Vector Concatenate/2
  Constant/1 -> Sum/1
  Vector Concatenate/1 -> Vector Concatenate1/2, Vector Concatenate1/1
  Demux/2 -> Trigonometric Function/1  "q2"
  Demux/1 -> Terminator/1
  Sum/1 -> M/1  "M"
  Vector Concatenate1/1 -> Gain/1
  xi1/1 -> Demux/1

== system Simulink_with_unkown_parameters_case/Matrix M(xi) approximation error 2/Matrix M(xi)  ==
  xi1 : Inport
  Constant : Constant  Value=[p1+p2+p4,p2;p2,p2+p5]
  Demux : Demux  Outputs=2
  Gain : Gain  Gain=[2*p3,p3;p3,0]
  Sum : Sum  Inputs=|++
  Terminator : Terminator
  Trigonometric Function : Trigonometry  Operator=cos
  Vector Concatenate : Concatenate  Mode=Multidimensional array
  Vector Concatenate1 : Concatenate  Mode=Multidimensional array  ConcatenateDimension=2
  M : Outport
  wires:
  xi1/1 -> Demux/1
  Vector Concatenate1/1 -> Gain/1
  Sum/1 -> M/1  "M"
  Demux/1 -> Terminator/1
  Demux/2 -> Trigonometric Function/1  "q2"
  Vector Concatenate/1 -> Vector Concatenate1/1, Vector Concatenate1/2
  Constant/1 -> Sum/1
  Trigonometric Function/1 -> Vector Concatenate/2, Vector Concatenate/1
  Gain/1 -> Sum/2

== system Simulink_with_unkown_parameters_case/Matrix M(xi) approximation error 3/Matrix M(xi)  ==
  xi1 : Inport
  Constant : Constant  Value=[p1+p2+p4,p2;p2,p2+p5]
  Demux : Demux  Outputs=2
  Gain : Gain  Gain=[2*p3,p3;p3,0]
  Sum : Sum  Inputs=|++
  Terminator : Terminator
  Trigonometric Function : Trigonometry  Operator=cos
  Vector Concatenate : Concatenate  Mode=Multidimensional array
  Vector Concatenate1 : Concatenate  Mode=Multidimensional array  ConcatenateDimension=2
  M : Outport
  wires:
  xi1/1 -> Demux/1
  Vector Concatenate1/1 -> Gain/1
  Sum/1 -> M/1  "M"
  Demux/1 -> Terminator/1
  Demux/2 -> Trigonometric Function/1  "q2"
  Vector Concatenate/1 -> Vector Concatenate1/1, Vector Concatenate1/2
  Constant/1 -> Sum/1
  Trigonometric Function/1 -> Vector Concatenate/2, Vector Concatenate/1
  Gain/1 -> Sum/2

== system Simulink_with_unkown_parameters_case/Matrix M(xi) approximation error 4/Matrix M(xi)  ==
  xi1 : Inport
  Constant : Constant  Value=[p1+p2+p4,p2;p2,p2+p5]
  Demux : Demux  Outputs=2
  Gain : Gain  Gain=[2*p3,p3;p3,0]
  Sum : Sum  Inputs=|++
  Terminator : Terminator
  Trigonometric Function : Trigonometry  Operator=cos
  Vector Concatenate : Concatenate  Mode=Multidimensional array
  Vector Concatenate1 : Concatenate  Mode=Multidimensional array  ConcatenateDimension=2
  M : Outport
  wires:
  Gain/1 -> Sum/2
  Trigonometric Function/1 -> Vector Concatenate/1, Vector Concatenate/2
  Constant/1 -> Sum/1
  Vector Concatenate/1 -> Vector Concatenate1/2, Vector Concatenate1/1
  Demux/2 -> Trigonometric Function/1  "q2"
  Demux/1 -> Terminator/1
  Sum/1 -> M/1  "M"
  Vector Concatenate1/1 -> Gain/1
  xi1/1 -> Demux/1

== system Simulink_with_unkown_parameters_case/planar 1/Jacobian matrix ==
  q : Inport
  Demux : Demux  Outputs=2
  Gain : Gain  Gain=-l1
  Gain1 : Gain  Gain=-l2
  Gain2 : Gain  Gain=l1
  Gain3 : Gain  Gain=l2
  Sum : Sum  Inputs=++|
  Sum1 : Sum  Inputs=|++
  Sum2 : Sum  Inputs=|++
  Trigonometric Function : Trigonometry
  Trigonometric Function1 : Trigonometry
  Trigonometric Function2 : Trigonometry  Operator=cos
  Trigonometric Function3 : Trigonometry  Operator=cos
  Vector Concatenate : Concatenate  Mode=Multidimensional array  ConcatenateDimension=2
  Vector Concatenate1 : Concatenate  Mode=Multidimensional array  ConcatenateDimension=2
  Vector Concatenate2 : Concatenate  Mode=Multidimensional array
  J(q) : Outport
  wires:
  Vector Concatenate2/1 -> J(q)/1
  Vector Concatenate/1 -> Vector Concatenate2/2
  Vector Concatenate1/1 -> Vector Concatenate2/1
  Sum2/1 -> Vector Concatenate/1  "J21"
  Sum1/1 -> Vector Concatenate1/1  "J11"
  Gain3/1 -> Vector Concatenate/2, Sum2/2  "J22"
  Gain2/1 -> Sum2/1
  Gain/1 -> Sum1/1
  Gain1/1 -> Sum1/2, Vector Concatenate1/2  "J12"
  Trigonometric Function2/1 -> Gain2/1
  Trigonometric Function3/1 -> Gain3/1
  Trigonometric Function1/1 -> Gain1/1
  Sum/1 -> Trigonometric Function3/1, Trigonometric Function1/1
  Demux/1 -> Trigonometric Function2/1, Trigonometric Function/1, Sum/1  "q1"
  Trigonometric Function/1 -> Gain/1
  Demux/2 -> Sum/2  "q2"
  q/1 -> Demux/1

== system Simulink_with_unkown_parameters_case/planar 1/Matrix C(q,dq)  ==
  q : Inport
  dq : Inport  Port=2
  Demux : Demux  Outputs=2
  Demux1 : Demux  Outputs=2
  Gain : Gain  Gain=[-p3,-p3;p3,0]
  Gain1 : Gain  Gain=[0,1;1,0]
  Gain2 : Gain  Gain=[1,0;0,0]
  Product : Product
  Sum : Sum
  Terminator : Terminator
  Trigonometric Function : Trigonometry
  Vector Concatenate : Concatenate  Mode=Multidimensional array
  Vector Concatenate1 : Concatenate  Mode=Multidimensional array  ConcatenateDimension=2
  C : Outport
  wires:
  Product/1 -> C/1
  Sum/1 -> Product/2
  Gain2/1 -> Sum/2
  Gain1/1 -> Sum/1
  Demux1/2 -> Gain2/1  "dq2"
  Demux1/1 -> Gain1/1  "dq1"
  dq/1 -> Demux1/1
  Gain/1 -> Product/1
  Trigonometric Function/1 -> Vector Concatenate/1, Vector Concatenate/2
  Vector Concatenate/1 -> Vector Concatenate1/2, Vector Concatenate1/1
  Demux/2 -> Trigonometric Function/1  "q2"
  Demux/1 -> Terminator/1
  Vector Concatenate1/1 -> Gain/1
  q/1 -> Demux/1

== system Simulink_with_unkown_parameters_case/planar 1/Matrix F ==
  Constant : Constant  Value=[p9,0;0,p10]
  F : Outport
  wires:
  Constant/1 -> F/1

== system Simulink_with_unkown_parameters_case/planar 1/Matrix G(q) ==
  q : Inport
  Demux : Demux  Outputs=2
  Gain : Gain  Gain=[p6,p7;0,p8]  Multiplication=Matrix(K*u)
  Mux : Mux  Inputs=2
  Sum : Sum  Inputs=++|
  Trigonometric Function : Trigonometry  Operator=cos
  Trigonometric Function1 : Trigonometry  Operator=cos
  G : Outport
  wires:
  Mux/1 -> Gain/1
  Trigonometric Function1/1 -> Mux/2
  Trigonometric Function/1 -> Mux/1
  Sum/1 -> Trigonometric Function1/1  "q1+q2"
  q/1 -> Demux/1
  Demux/1 -> Trigonometric Function/1, Sum/1  "q1"
  Demux/2 -> Sum/2  "q2"
  Gain/1 -> G/1

== system Simulink_with_unkown_parameters_case/planar 1/Matrix M(q)  ==
  q : Inport
  Constant : Constant  Value=[p1+p2+p4,p2;p2,p2+p5]
  Demux : Demux  Outputs=2
  Gain : Gain  Gain=[2*p3,p3;p3,0]
  Sum : Sum  Inputs=|++
  Terminator : Terminator
  Trigonometric Function : Trigonometry  Operator=cos
  Vector Concatenate : Concatenate  Mode=Multidimensional array
  Vector Concatenate1 : Concatenate  Mode=Multidimensional array  ConcatenateDimension=2
  M : Outport
  wires:
  q/1 -> Demux/1
  Vector Concatenate1/1 -> Gain/1
  Sum/1 -> M/1  "M"
  Demux/1 -> Terminator/1
  Demux/2 -> Trigonometric Function/1  "q2"
  Vector Concatenate/1 -> Vector Concatenate1/1, Vector Concatenate1/2
  Constant/1 -> Sum/1
  Trigonometric Function/1 -> Vector Concatenate/2, Vector Concatenate/1
  Gain/1 -> Sum/2

== system Simulink_with_unkown_parameters_case/planar 1/forward kinematics ==
  q : Inport
  Constant : Constant  Value=x0
  Demux : Demux  Outputs=2
  Gain : Gain  Gain=l1
  Gain1 : Gain  Gain=l2
  Gain2 : Gain  Gain=l1
  Gain3 : Gain  Gain=l2
  Mux : Mux  Inputs=2
  Sum : Sum  Inputs=++|
  Sum1 : Sum  Inputs=++|
  Sum2 : Sum  Inputs=|++
  Sum3 : Sum  Inputs=|++
  Trigonometric Function : Trigonometry  Operator=cos
  Trigonometric Function1 : Trigonometry  Operator=cos
  Trigonometric Function2 : Trigonometry
  Trigonometric Function3 : Trigonometry
  x : Outport
  wires:
  Constant/1 -> Sum3/2
  Sum3/1 -> x/1
  Sum2/1 -> Mux/2
  Sum1/1 -> Mux/1
  Gain3/1 -> Sum2/2
  Gain2/1 -> Sum2/1
  Gain/1 -> Sum1/1
  Gain1/1 -> Sum1/2
  Trigonometric Function2/1 -> Gain2/1
  Trigonometric Function3/1 -> Gain3/1
  Trigonometric Function1/1 -> Gain1/1
  Sum/1 -> Trigonometric Function3/1, Trigonometric Function1/1
  Demux/1 -> Trigonometric Function2/1, Trigonometric Function/1, Sum/1  "q1"
  Trigonometric Function/1 -> Gain/1
  Demux/2 -> Sum/2  "q2"
  Mux/1 -> Sum3/1
  q/1 -> Demux/1

== system Simulink_with_unkown_parameters_case/planar 2/Jacobian matrix ==
  q : Inport
  Demux : Demux  Outputs=2
  Gain : Gain  Gain=-l1
  Gain1 : Gain  Gain=-l2
  Gain2 : Gain  Gain=l1
  Gain3 : Gain  Gain=l2
  Sum : Sum  Inputs=++|
  Sum1 : Sum  Inputs=|++
  Sum2 : Sum  Inputs=|++
  Trigonometric Function : Trigonometry
  Trigonometric Function1 : Trigonometry
  Trigonometric Function2 : Trigonometry  Operator=cos
  Trigonometric Function3 : Trigonometry  Operator=cos
  Vector Concatenate : Concatenate  Mode=Multidimensional array  ConcatenateDimension=2
  Vector Concatenate1 : Concatenate  Mode=Multidimensional array  ConcatenateDimension=2
  Vector Concatenate2 : Concatenate  Mode=Multidimensional array
  J(q) : Outport
  wires:
  Vector Concatenate2/1 -> J(q)/1
  Vector Concatenate/1 -> Vector Concatenate2/2
  Vector Concatenate1/1 -> Vector Concatenate2/1
  Sum2/1 -> Vector Concatenate/1  "J21"
  Sum1/1 -> Vector Concatenate1/1  "J11"
  Gain3/1 -> Vector Concatenate/2, Sum2/2  "J22"
  Gain2/1 -> Sum2/1
  Gain/1 -> Sum1/1
  Gain1/1 -> Sum1/2, Vector Concatenate1/2  "J12"
  Trigonometric Function2/1 -> Gain2/1
  Trigonometric Function3/1 -> Gain3/1
  Trigonometric Function1/1 -> Gain1/1
  Sum/1 -> Trigonometric Function3/1, Trigonometric Function1/1
  Demux/1 -> Trigonometric Function2/1, Trigonometric Function/1, Sum/1  "q1"
  Trigonometric Function/1 -> Gain/1
  Demux/2 -> Sum/2  "q2"
  q/1 -> Demux/1

== system Simulink_with_unkown_parameters_case/planar 2/Matrix C(q,dq)  ==
  q : Inport
  dq : Inport  Port=2
  Demux : Demux  Outputs=2
  Demux1 : Demux  Outputs=2
  Gain : Gain  Gain=[-p3,-p3;p3,0]
  Gain1 : Gain  Gain=[0,1;1,0]
  Gain2 : Gain  Gain=[1,0;0,0]
  Product : Product
  Sum : Sum
  Terminator : Terminator
  Trigonometric Function : Trigonometry
  Vector Concatenate : Concatenate  Mode=Multidimensional array
  Vector Concatenate1 : Concatenate  Mode=Multidimensional array  ConcatenateDimension=2
  C : Outport
  wires:
  Product/1 -> C/1
  Sum/1 -> Product/2
  Gain2/1 -> Sum/2
  Gain1/1 -> Sum/1
  Demux1/2 -> Gain2/1  "dq2"
  Demux1/1 -> Gain1/1  "dq1"
  dq/1 -> Demux1/1
  Gain/1 -> Product/1
  Trigonometric Function/1 -> Vector Concatenate/1, Vector Concatenate/2
  Vector Concatenate/1 -> Vector Concatenate1/2, Vector Concatenate1/1
  Demux/2 -> Trigonometric Function/1  "q2"
  Demux/1 -> Terminator/1
  Vector Concatenate1/1 -> Gain/1
  q/1 -> Demux/1

== system Simulink_with_unkown_parameters_case/planar 2/Matrix F ==
  Constant : Constant  Value=[p9,0;0,p10]
  F : Outport
  wires:
  Constant/1 -> F/1

== system Simulink_with_unkown_parameters_case/planar 2/Matrix G(q) ==
  q : Inport
  Demux : Demux  Outputs=2
  Gain : Gain  Gain=[p6,p7;0,p8]  Multiplication=Matrix(K*u)
  Mux : Mux  Inputs=2
  Sum : Sum  Inputs=++|
  Trigonometric Function : Trigonometry  Operator=cos
  Trigonometric Function1 : Trigonometry  Operator=cos
  G : Outport
  wires:
  Mux/1 -> Gain/1
  Trigonometric Function1/1 -> Mux/2
  Trigonometric Function/1 -> Mux/1
  Sum/1 -> Trigonometric Function1/1  "q1+q2"
  q/1 -> Demux/1
  Demux/1 -> Trigonometric Function/1, Sum/1  "q1"
  Demux/2 -> Sum/2  "q2"
  Gain/1 -> G/1

== system Simulink_with_unkown_parameters_case/planar 2/Matrix M(q)  ==
  q : Inport
  Constant : Constant  Value=[p1+p2+p4,p2;p2,p2+p5]
  Demux : Demux  Outputs=2
  Gain : Gain  Gain=[2*p3,p3;p3,0]
  Sum : Sum  Inputs=|++
  Terminator : Terminator
  Trigonometric Function : Trigonometry  Operator=cos
  Vector Concatenate : Concatenate  Mode=Multidimensional array
  Vector Concatenate1 : Concatenate  Mode=Multidimensional array  ConcatenateDimension=2
  M : Outport
  wires:
  q/1 -> Demux/1
  Vector Concatenate1/1 -> Gain/1
  Sum/1 -> M/1  "M"
  Demux/1 -> Terminator/1
  Demux/2 -> Trigonometric Function/1  "q2"
  Vector Concatenate/1 -> Vector Concatenate1/1, Vector Concatenate1/2
  Constant/1 -> Sum/1
  Trigonometric Function/1 -> Vector Concatenate/2, Vector Concatenate/1
  Gain/1 -> Sum/2

== system Simulink_with_unkown_parameters_case/planar 2/forward kinematics ==
  q : Inport
  Constant : Constant  Value=x0
  Demux : Demux  Outputs=2
  Gain : Gain  Gain=l1
  Gain1 : Gain  Gain=l2
  Gain2 : Gain  Gain=l1
  Gain3 : Gain  Gain=l2
  Mux : Mux  Inputs=2
  Sum : Sum  Inputs=++|
  Sum1 : Sum  Inputs=++|
  Sum2 : Sum  Inputs=|++
  Sum3 : Sum  Inputs=|++
  Trigonometric Function : Trigonometry  Operator=cos
  Trigonometric Function1 : Trigonometry  Operator=cos
  Trigonometric Function2 : Trigonometry
  Trigonometric Function3 : Trigonometry
  x : Outport
  wires:
  Constant/1 -> Sum3/2
  Sum3/1 -> x/1
  Sum2/1 -> Mux/2
  Sum1/1 -> Mux/1
  Gain3/1 -> Sum2/2
  Gain2/1 -> Sum2/1
  Gain/1 -> Sum1/1
  Gain1/1 -> Sum1/2
  Trigonometric Function2/1 -> Gain2/1
  Trigonometric Function3/1 -> Gain3/1
  Trigonometric Function1/1 -> Gain1/1
  Sum/1 -> Trigonometric Function3/1, Trigonometric Function1/1
  Demux/1 -> Trigonometric Function2/1, Trigonometric Function/1, Sum/1  "q1"
  Trigonometric Function/1 -> Gain/1
  Demux/2 -> Sum/2  "q2"
  Mux/1 -> Sum3/1
  q/1 -> Demux/1
